simulink model "QuadcopterAF"  (R2023b)
settings: Solver=VariableStepAuto  StartTime=0.0  StopTime=30  RelTol=1e-3
libraries: fl_lib x14, nesl_utility x3
settings Model: Creator=bneiswan  LastModifiedBy=ntrica

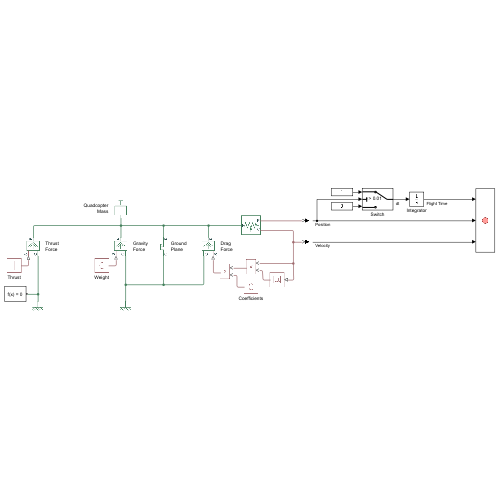
[thumbnail: Simulink's stored preview of the top-level diagram]
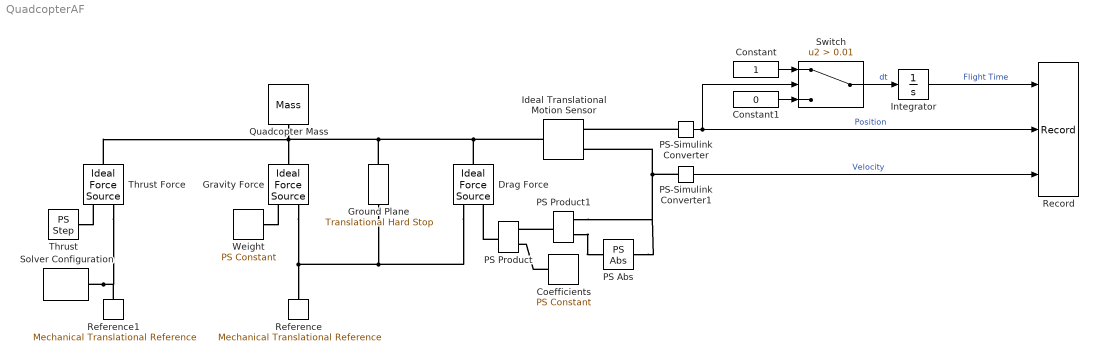
== system QuadcopterAF ==
  Coefficients : fl_lib/Physical Signals/Sources/PS Constant  constant=-1/2*1.225*1.1*0.006 N/(m/s)^2
  Constant : Constant
  Constant1 : Constant  Value=0
  Drag Force : fl_lib/Mechanical/Mechanical Sources/Ideal Force Source
  Gravity Force : fl_lib/Mechanical/Mechanical Sources/Ideal Force Source
  Ground Plane : fl_lib/Mechanical/Translational Elements/Translational Hard Stop  upper_bnd=inf m  lower_bnd=0 m  model=simscape.enum.hardstop.smooth  stiff_up=1e6 N/m  stiff_low=200 N/m  D_up=150 N*s/m  D_low=150 N*s/m  transition=0.1 mm  coeff_rest=0.7  v_tol=0.001 m/s  f_tol=0.001 N  v_specify=off  v_priority=None  v=0 m/s  v_nominal_specify=off  v_nominal_unit=m/s  v_nominal_value=1  f_specify=off  f_priority=None  f=0 N  f_nominal_specify=off  f_nominal_unit=N  f_nominal_value=1  x_specify=off  x_priority=High  x=0 m  x_nominal_specify=off  x_nominal_unit=m  x_nominal_value=1  M_specify=off  M_priority=None  M=0
  Ideal Translational Motion Sensor : fl_lib/Mechanical/Mechanical Sensors/Ideal Translational Motion Sensor  reference=foundation.enum.MeasurementReference.absolute  acceleration_port=false  velocity_port=true  position_port=true  offset=0 m
      settings: InternalSimscapePortConfiguration="{\"Bottom\":[],\"Left\":[{\"id\":\"R\",\"label\":\"R\",\"type\":\"foundation.mechanical.translational.translational\"}],\"Right\":[{\"id\":\"V\",\"label\":\"V\",\"type\":\"output\"},{\"id\":\"P\",\"label\":\"P\",\"type\":\"output\"}],\"Top\":[]}"
  Integrator : Integrator
  PS Abs : fl_lib/Physical Signals/Nonlinear Operators/PS Abs
      settings: InternalSimscapePortConfiguration="{\"Bottom\":[],\"Left\":[{\"id\":\"I\",\"label\":\"\",\"type\":\"input\"}],\"Right\":[{\"id\":\"O\",\"label\":\"\",\"type\":\"output\"}],\"Top\":[]}"
  PS Product : fl_lib/Physical Signals/Functions/PS Product
  PS Product1 : fl_lib/Physical Signals/Functions/PS Product
  PS-Simulink Converter : nesl_utility/PS-Simulink Converter  PhysicalDomain=network_engine_domain  SubClassName=ps_output  LeftPortType=input  RightPortType=output  PseudoPeriodic=off  Frequencies=[]  VectorFormat=inherit  Unit=m  AffineConversion=off
  PS-Simulink Converter1 : nesl_utility/PS-Simulink Converter  PhysicalDomain=network_engine_domain  SubClassName=ps_output  LeftPortType=input  RightPortType=output  PseudoPeriodic=off  Frequencies=[]  VectorFormat=inherit  Unit=km/hr  AffineConversion=off
  Quadcopter Mass : fl_lib/Mechanical/Translational Elements/Mass  mass=0.07 kg  num_ports=foundation.enum.numPorts2.one  v_specify=off  v_priority=High  v=0 m/s  v_nominal_specify=off  v_nominal_unit=m/s  v_nominal_value=1  f_specify=off  f_priority=None  f=0 N  f_nominal_specify=off  f_nominal_unit=N  f_nominal_value=1
  Record : Record  FileSettingsInternal="{\"entries\":[{\"content\":{\"excelSettings\":{\"content\":{},\"type\":\"Streamout.ExcelSettings\"}},\"type\":\"Streamout.FileSettingStorage\",\"uuid\":\"\"}],\"packageUris\":[\"http:\\/\\/schema.mathworks.com\\/mf0\\/streamout_blocks\\/R2020a\"],\"version\":\"1.0\"}"  SignalsInternal="{\"entries\":[{\"content\":{\"signals\":[{\"content\":{\"blockPath\":[],\"dimensions\":[1,1],\"domain\":\"\",\"lineColor\":\"#22b573\",\"plots\":[1],\"port\":1,\"signalID\":247,\"signalName\":\"Flight Time\"},\"type\":\"RecordBlkView.Signal\",\"uuid\":\"\"},{\"content\":{\"blockPath\":[],\"dimensions\":[1,1],\"domain\":\"\",\"lineColor\":\"#0072bd\",\"plots\":[1],\"port\":2,\"signalID\":250,\"signalName\":\"Position\"},\"type\":\"RecordBlkView.Signal\",\"uuid\":\"\"},{\"content\":{\"blockPath\":[],\"dimensions\":[1,1],\"domain\":\"\",\"lineColor\":\"#d95319\",\"plots\":[1],\"port\":3,\"signalID\":253,\"signalName\":\"Velocity\"},\"type\":\"RecordBlkView.Signal\",\"uuid\":\"\"}]},\"type\":\"RecordBlkView.InputSignals\",\"uuid\":\"\"}],\"packageUris\":[\"http:\\/\\/schema.mathworks.com\\/mf0\\/streamout_blocks\\/R2020a\"],\"version\":\"1.0\"}"  VisualizationBindings="{\"sparklinesplugin\":{\"info\":[{\"bindingParametersList\":[],\"subplotID\":1}]}}"
  Reference : fl_lib/Mechanical/Translational Elements/Mechanical Translational Reference
  Reference1 : fl_lib/Mechanical/Translational Elements/Mechanical Translational Reference
  Solver Configuration : nesl_utility/Solver Configuration  PhysicalDomain=network_engine_domain  SubClassName=solver  LeftPortType=input  RightPortType=generic  Tones=[]  Harmonics=[]  SimulateNoise=off  Profile=off  UseLocalSampling=off  EnableSwitchedLinearOptims=on  FrequencyDomain=off  UseCCode=off  RelTol=0.001  AbsTol=0.001  MinStep=1e-09  ToWorkspace=off  RevertToSquareIcSolve=off  NumHomotopyIterations=100  PhasorMode=off  PhasorModeNumHarmonics=1  ConsistencySolver=NEWTON_XTOL_AFTER_FTOL  IndexReductionMethod=DerivativeReplacement  DoDC=off  ResidualTolerance=1e-09  ConsistencyTolSource=GLOBAL  ConsistencyAbsTol=0.001  ConsistencyRelTol=0.001  ConsistencyTolFactor=0.001  UseLocalSolver=off  LocalSolverChoice=NE_BACKWARD_EULER_ADVANCER  ResolveIndetEquations=on  FunctionEvalNumThread=1  LocalSolverSampleTime=0.001  DoFixedCost=off  MaxNonlinIter=3  MaxModeIter=2  ComputeImpulses=off  ImpulseIterations=2  LinearAlgebra=auto  LinearAlgebraNumThread=0  EquationFormulation=NE_TIME_EF  DelaysMemoryBudget=1024  AutomaticFiltering=on  FilteringTimeConstant=0.001  PartitionStorageMethod=AS_NEEDED  PartitionMemoryBudget=1024  PartitionMethod=ROBUST  MultibodyUseLocalSolver=off  MultibodyLocalSolverChoice=ODE1  MultibodyLocalSolverSampleTime=0.001
  Switch : Switch  Criteria=u2 > Threshold  Threshold=0.01  SaturateOnIntegerOverflow=off  InputSameDT=off
  Thrust : fl_lib/Physical Signals/Sources/PS Step  step_time=15 s  initial_value=0.8 N  final_value=0 N
  Thrust Force : fl_lib/Mechanical/Mechanical Sources/Ideal Force Source
  Weight : fl_lib/Physical Signals/Sources/PS Constant  constant=-0.07*9.81 N
  wires:
  Constant/1 -> Switch/1
  Switch/1 -> Integrator/1  "dt"
  Constant1/1 -> Switch/3
  PS-Simulink Converter1/1 -> Record/3  "Velocity"
  PS-Simulink Converter/1 -> Record/2, Switch/2  "Position"
  Integrator/1 -> Record/1  "Flight Time"
  connections:
  PS-Simulink Converter1/LConn1 -- Ideal Translational Motion Sensor/RConn1 -- PS Product1/LConn1 -- PS Abs/LConn1
  Drag Force/LConn1 -- Quadcopter Mass/LConn1 -- Gravity Force/LConn1 -- Thrust Force/LConn1 -- Ground Plane/LConn1 -- Ideal Translational Motion Sensor/LConn1
  Solver Configuration/RConn1 -- Thrust Force/RConn2 -- Reference1/LConn1
  Ground Plane/RConn1 -- Gravity Force/RConn2 -- Reference/LConn1 -- Drag Force/RConn2
  Thrust/RConn1 -- Thrust Force/RConn1
  PS Product1/LConn2 -- PS Abs/RConn1
  PS-Simulink Converter/LConn1 -- Ideal Translational Motion Sensor/RConn2
  Coefficients/RConn1 -- PS Product/LConn2
  PS Product/RConn1 -- Drag Force/RConn1
  PS Product1/RConn1 -- PS Product/LConn1
  Weight/RConn1 -- Gravity Force/RConn1
